simulink model "nmpc_sim"  (R2022a)
settings: Solver=VariableStepAuto  StartTime=0.0  StopTime=10.0  RelTol=1e-3
values from neighbouring files (symbols this model uses):
  Ts = 0.5    [nmpc_matlab.m]    (also in nmpc_test.m = 0.1)
libraries: mpclib x1
settings Model: Creator=charl  LastModifiedBy=charl

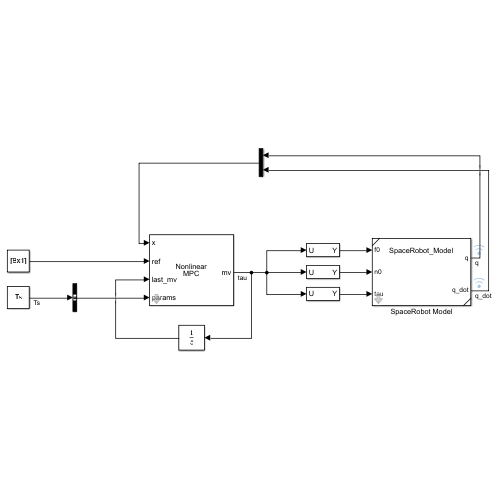
[thumbnail: Simulink's stored preview of the top-level diagram]
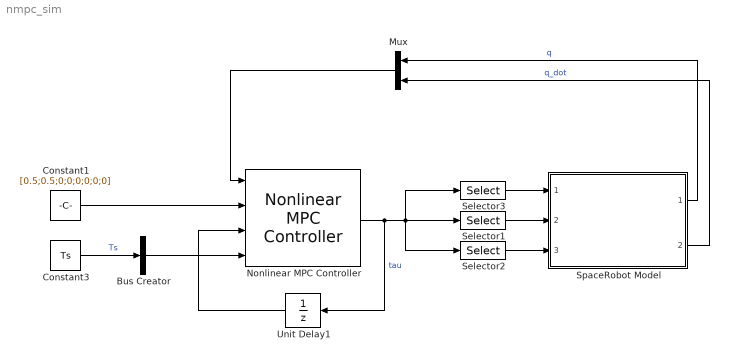
== system nmpc_sim ==
  Bus Creator : BusCreator  Inputs=1  OutDataTypeStr=Bus: myBusObject  NonVirtualBus=on
      settings: InheritFromInputs=off
  Constant1 : Constant  Value=[0.5;0.5;0;0;0;0;0;0]
  Constant3 : Constant  Value=Ts
  Mux : Mux  Inputs=2
  Nonlinear MPC Controller : mpclib/Nonlinear MPC Controller  SCDEnableBlockLinearizationSpecification=on  nlmpcobj=nlobj  UseObjectTs=on  UseMEX=off  md_enabled=off  mvtarget_enabled=off  param_enabled=on  cost_enabled=off  mvseq_enabled=off  stateseq_enabled=off  ovseq_enabled=off  slack_enabled=off  status_enabled=off  ov_min=off  ov_max=off  mv_min=off  mv_max=off  mvrate_min=off  mvrate_max=off  state_min=off  state_max=off  ov_weight=off  mv_weight=off  mvrate_weight=off  ecr_weight=off  nlp_initialize=off
  Selector1 : Selector  IndexOptions=Index vector (dialog)  Indices=[1:6]  OutputSizes=1
  Selector2 : Selector  IndexOptions=Index vector (dialog)  Indices=[1:6]  OutputSizes=1
  Selector3 : Selector  IndexOptions=Index vector (dialog)  Indices=[1:6]  OutputSizes=1
  SpaceRobot Model : Subsystem  ReferencedSubsystem=SpaceRobot_Model  spaceRobot=sr
  Unit Delay1 : UnitDelay  SampleTime=-1  HasFrameUpgradeWarning=on
  wires:
  Nonlinear MPC Controller/1 -> Unit Delay1/1, Selector3/1, Selector2/1, Selector1/1  "tau"
  Selector2/1 -> SpaceRobot Model/3
  Selector1/1 -> SpaceRobot Model/2
  Selector3/1 -> SpaceRobot Model/1
  Unit Delay1/1 -> Nonlinear MPC Controller/3
  Constant1/1 -> Nonlinear MPC Controller/2
  Mux/1 -> Nonlinear MPC Controller/1
  SpaceRobot Model/2 -> Mux/2  "q_dot"
  SpaceRobot Model/1 -> Mux/1  "q"
  Bus Creator/1 -> Nonlinear MPC Controller/4
  Constant3/1 -> Bus Creator/1  "Ts"
